simulink model "carritos_sobre_carrito"  (R2017b)
settings: Solver=ode45  StartTime=0.0  StopTime=3000  MaxStep=0.001  RelTol=1e-6  AbsTol=1e-6
settings Model: Creator=Erick  LastModifiedBy=Erick

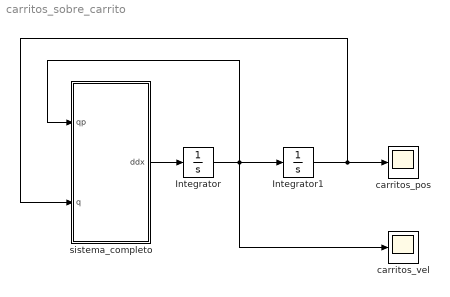
== system carritos_sobre_carrito ==
  Integrator : Integrator  InitialCondition=[0 0 0 0 0]
  Integrator1 : Integrator  InitialCondition=[3e-3 0 -2e-3 0 0]
  carritos_pos : Scope
  carritos_vel : Scope
  sistema_completo : MATLAB Function  TreatAsAtomicUnit=on
  wires:
  Integrator1/1 -> carritos_pos/1, sistema_completo/2(q)
  sistema_completo/1(ddx) -> Integrator/1
  Integrator/1 -> Integrator1/1, carritos_vel/1, sistema_completo/1(qp)

== matlab function carritos_sobre_carrito/sistema_completo ==
  data: qp input; q input; ddx output
function ddx = fcn(qp,q)
% estados
x1 = q(1);
x2 = q(2);
x3 = q(3);
x4 = q(4);
x5 = q(5);

x1p = qp(1);
x2p = qp(2);
x3p = qp(3);
x4p = qp(4);
x5p = qp(5);

% parametros
k1 = 37.10; %Nm
k2 = 37.10; %Nm
k3 = 37.10; %Nm
k4 = 37.10; %Nm
k5 = 388.71; %Nm

% b1 = 0.05;
% b2 = 0.05;
% b3 = 0.05;
% b4 = 0.05;
b5 = 3.2656;
% b5 = 0.05;
% b5 = b5_sim;

b1 = 0;
b2 = 0;
b3 = 0;
b4 = 0;
% b5 = 0;

m1 = 0.21; %kg
m2 = 0.21; %kg
m3 = 0.21; %kg
m4 = 0.21; %kg
m5 = 20; %kg %m5=<0.8 contra-fase , m5>0.8 en-fase + CI
% m5 = m5_sim;

%ganancias de control
% k_1 = 0.5;
% k_2 = 1.5;
% k_3 = 0.5;
% k_4 = 1.5;

V = 125.0982; % lambda
H = 7.835e-4;

% temrminos del oscilador
h1 = (1/2)*m1*x1p^2+(1/2)*k1*x1^2;
h2 = (1/2)*m3*x3p^2+(1/2)*k3*x3^2;

u1 = -V*(h1-H)*x1p;
u2 = -V*(h2-H)*x3p;

% u1 = k_1*x1+k_2*x2+k_3*x1p+k_4*x2p; % carrito 1
% u2 = k_1*x3+k_2*x4+k_3*x3p+k_4*x4p; % carrito 2

ddx = [(1/m1)*(-k1*(x1-x5)+k2*(x2-x1)-b1*(x1p-x5p)-b2*(x1p-x2p)+u1);
       (1/m2)*(-k2*(x2-x1)-b2*(x2p-x1p));
       (1/m3)*(-k3*(x3-x5)+k4*(x4-x3)-b3*(x3p-x5p)-b4*(x3p-x4p)+u2);
       (1/m4)*(-k4*(x4-x3)-b4*(x4p-x3p));
       (1/m5)*(k1*(x1-x5)+k3*(x3-x5)-k5*(x5)-b5*(x5p)-u1-u2)
       ];
